simulink model "Induction_Motor_Simulation"  (R2021b)
settings: Solver=ode45  StartTime=0.0  StopTime=1  MinStep=1e-5  RelTol=1e-6
undefined symbols (not defined in the file): B, f_supply, J, L_ms, Lr_diag, Lr_non_diag, Ls_diag, Ls_non_diag, P, r_r, r_s, T_L, V_as, V_bs, V_cs
settings Model: Creator=pghat  LastModifiedBy=pghat
settings DebuggingCC: AlgebraicLoopMsg=none

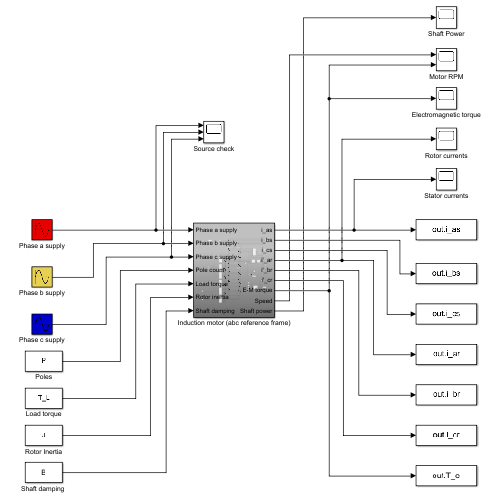
[thumbnail: Simulink's stored preview of the top-level diagram]
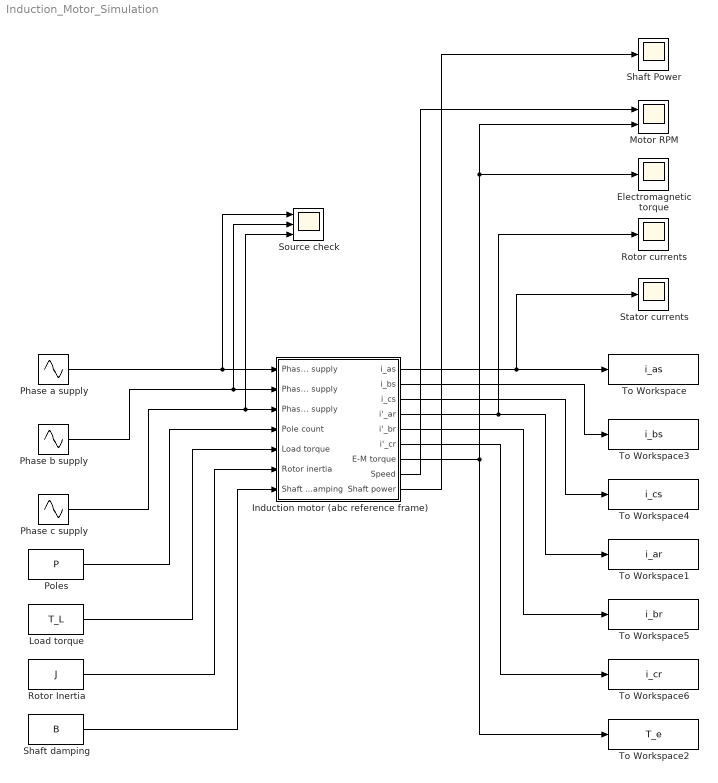
== system Induction_Motor_Simulation ==
  Electromagnetic torque : Scope
  Induction motor (abc reference frame) : Subsystem
  Load torque : Constant  Value=T_L
  Motor RPM : Scope  NumInputPorts=2
  Phase a supply : Sin  Amplitude=V_as  Frequency=f_supply  Phase=pi/2  SampleTime=0
  Phase b supply : Sin  Amplitude=V_bs  Frequency=f_supply  Phase=((2*pi)/3)+(pi/2)  SampleTime=0
  Phase c supply : Sin  Amplitude=V_cs  Frequency=f_supply  Phase=(-(2*pi)/3)+(pi/2)  SampleTime=0
  Poles : Constant  Value=P
  Rotor Inertia : Constant  Value=J
  Rotor currents : Scope
  Shaft Power : Scope
  "Shaft damping " : Constant  Value=B
  Source check : Scope  NumInputPorts=3
  Stator currents : Scope
  To Workspace : ToWorkspace  VariableName=i_as  SampleTime=-1
  To Workspace1 : ToWorkspace  VariableName=i_ar  SampleTime=-1
  To Workspace2 : ToWorkspace  VariableName=T_e  SampleTime=-1
  To Workspace3 : ToWorkspace  VariableName=i_bs  SampleTime=-1
  To Workspace4 : ToWorkspace  VariableName=i_cs  SampleTime=-1
  To Workspace5 : ToWorkspace  VariableName=i_br  SampleTime=-1
  To Workspace6 : ToWorkspace  VariableName=i_cr  SampleTime=-1
  wires:
  Poles/1 -> Induction motor (abc reference frame)/4(Pole count)
  Induction motor (abc reference frame)/4(i'_ar) -> To Workspace1/1, Rotor currents/1
  Induction motor (abc reference frame)/1(i_as) -> To Workspace/1, Stator currents/1
  Induction motor (abc reference frame)/7(E-M torque) -> To Workspace2/1, Motor RPM/2, Electromagnetic torque/1
  Phase a supply/1 -> Source check/1, Induction motor (abc reference frame)/1(Phase a supply)
  Phase b supply/1 -> Source check/2, Induction motor (abc reference frame)/2(Phase b supply)
  Phase c supply/1 -> Source check/3, Induction motor (abc reference frame)/3(Phase c supply)
  Rotor Inertia/1 -> Induction motor (abc reference frame)/6(Rotor inertia)
  Induction motor (abc reference frame)/8(Speed) -> Motor RPM/1
  Load torque/1 -> Induction motor (abc reference frame)/5(Load torque)
  "Shaft damping "/1 -> Induction motor (abc reference frame)/7(Shaft damping)
  Induction motor (abc reference frame)/2(i_bs) -> To Workspace3/1
  Induction motor (abc reference frame)/3(i_cs) -> To Workspace4/1
  Induction motor (abc reference frame)/5(i'_br) -> To Workspace5/1
  Induction motor (abc reference frame)/6(i'_cr) -> To Workspace6/1
  Induction motor (abc reference frame)/9(Shaft power) -> Shaft Power/1

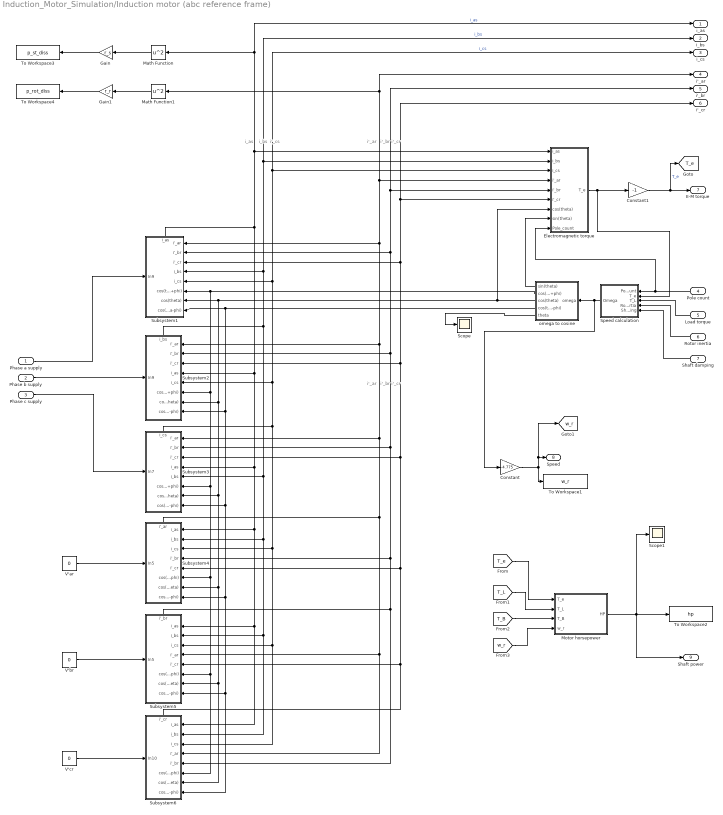
== system Induction_Motor_Simulation/Induction motor (abc reference frame) ==
  note: i'_ar
  note: i'_br
  note: i'_cr
  note: i_as
  note: i_bs
  note: i'_cs
  note: i'_br
  note: i'_ar
  note: i'_cr
  Phase a supply : Inport
  Phase b supply : Inport  Port=2
  Phase c supply : Inport  Port=3
  Pole count : Inport  Port=4
  Load torque : Inport  Port=5
  Rotor inertia : Inport  Port=6
  Shaft damping : Inport  Port=7
  Constant : Gain  Gain=-4.775
  Constant1 : Gain  Gain=-1
  Electromagnetic torque : Subsystem
  Gain : Gain  Gain=r_s
  Gain1 : Gain  Gain=r_r
  Math Function : Math  Operator=square  SaturateOnIntegerOverflow=on
  Math Function1 : Math  Operator=square  SaturateOnIntegerOverflow=on
  Motor horsepower : Subsystem
  Scope : Scope
  Scope1 : Scope
  Speed calculation : Subsystem
  Subsystem1 : Subsystem
      settings: PortSchema="{\"entries\":[{\"content\":{\"sides\":[{\"content\":{\"connectorIds\":[\"In1\",\"In2\",\"In3\",\"In4\",\"In5\",\"In6\",\"In7\",\"In8\"]},\"type\":\"ConnectorPlacement.EquallySpacedRectSide\",\"uuid\":\"ef07c968-7ee2-485d-9f10-a51b04dcb3ba\"},{\"content\":{\"connectorIds\":[\"In9\"],\"side\":\"RIGHT\"},\"type\":\"ConnectorPlacement.EquallySpacedRectSide\",\"uuid\":\"1cfd75a1-6326-417f-a91d-cffa3dd273c8\"},{\"content\":{\"connectorIds\":[\"Out1\"],\"side\":\"TOP\"},\"type\":\"ConnectorPlacement.EquallySpacedRectSide\",\"uuid\":\"a404849e-3712-479f-a728-f0b6851758dc\"}]},\"type\":\"ConnectorPlacement.EquallySpacedConnector\",\"uuid\":\"81e44c3d-c841-4212-bb95-4a45c20bd008\"}],\"packageUris\":[\"http://schema.mathworks.com/mf0/Connector/R2020b\"],\"version\":\"1.0\"}"
  Subsystem2 : Subsystem
      settings: PortSchema="{\"entries\":[{\"content\":{\"sides\":[{\"content\":{\"connectorIds\":[\"In1\",\"In2\",\"In3\",\"In4\",\"In5\",\"In6\",\"In7\",\"In8\"]},\"type\":\"ConnectorPlacement.EquallySpacedRectSide\",\"uuid\":\"ef07c968-7ee2-485d-9f10-a51b04dcb3ba\"},{\"content\":{\"connectorIds\":[\"In9\"],\"side\":\"RIGHT\"},\"type\":\"ConnectorPlacement.EquallySpacedRectSide\",\"uuid\":\"1cfd75a1-6326-417f-a91d-cffa3dd273c8\"},{\"content\":{\"connectorIds\":[\"Out1\"],\"side\":\"TOP\"},\"type\":\"ConnectorPlacement.EquallySpacedRectSide\",\"uuid\":\"a404849e-3712-479f-a728-f0b6851758dc\"}]},\"type\":\"ConnectorPlacement.EquallySpacedConnector\",\"uuid\":\"81e44c3d-c841-4212-bb95-4a45c20bd008\"}],\"packageUris\":[\"http://schema.mathworks.com/mf0/Connector/R2020b\"],\"version\":\"1.0\"}"
  Subsystem3 : Subsystem
      settings: PortSchema="{\"entries\":[{\"content\":{\"sides\":[{\"content\":{\"connectorIds\":[\"In1\",\"In2\",\"In3\",\"In4\",\"In5\",\"In6\",\"In7\",\"In8\"]},\"type\":\"ConnectorPlacement.EquallySpacedRectSide\",\"uuid\":\"ef07c968-7ee2-485d-9f10-a51b04dcb3ba\"},{\"content\":{\"connectorIds\":[\"In9\"],\"side\":\"RIGHT\"},\"type\":\"ConnectorPlacement.EquallySpacedRectSide\",\"uuid\":\"1cfd75a1-6326-417f-a91d-cffa3dd273c8\"},{\"content\":{\"connectorIds\":[\"Out1\"],\"side\":\"TOP\"},\"type\":\"ConnectorPlacement.EquallySpacedRectSide\",\"uuid\":\"a404849e-3712-479f-a728-f0b6851758dc\"}]},\"type\":\"ConnectorPlacement.EquallySpacedConnector\",\"uuid\":\"81e44c3d-c841-4212-bb95-4a45c20bd008\"}],\"packageUris\":[\"http://schema.mathworks.com/mf0/Connector/R2020b\"],\"version\":\"1.0\"}"
  Subsystem4 : Subsystem
      settings: PortSchema="{\"entries\":[{\"content\":{\"sides\":[{\"content\":{\"connectorIds\":[\"In1\",\"In2\",\"In3\",\"In4\",\"In5\",\"In6\",\"In7\",\"In8\"]},\"type\":\"ConnectorPlacement.EquallySpacedRectSide\",\"uuid\":\"ef07c968-7ee2-485d-9f10-a51b04dcb3ba\"},{\"content\":{\"connectorIds\":[\"In9\"],\"side\":\"RIGHT\"},\"type\":\"ConnectorPlacement.EquallySpacedRectSide\",\"uuid\":\"1cfd75a1-6326-417f-a91d-cffa3dd273c8\"},{\"content\":{\"connectorIds\":[\"Out1\"],\"side\":\"TOP\"},\"type\":\"ConnectorPlacement.EquallySpacedRectSide\",\"uuid\":\"a404849e-3712-479f-a728-f0b6851758dc\"}]},\"type\":\"ConnectorPlacement.EquallySpacedConnector\",\"uuid\":\"81e44c3d-c841-4212-bb95-4a45c20bd008\"}],\"packageUris\":[\"http://schema.mathworks.com/mf0/Connector/R2020b\"],\"version\":\"1.0\"}"
  Subsystem5 : Subsystem
      settings: PortSchema="{\"entries\":[{\"content\":{\"sides\":[{\"content\":{\"connectorIds\":[\"In1\",\"In2\",\"In3\",\"In4\",\"In5\",\"In6\",\"In7\",\"In8\"]},\"type\":\"ConnectorPlacement.EquallySpacedRectSide\",\"uuid\":\"0210d93f-9c3f-4c48-b905-c827d03e93dd\"},{\"content\":{\"connectorIds\":[\"In9\"],\"side\":\"RIGHT\"},\"type\":\"ConnectorPlacement.EquallySpacedRectSide\",\"uuid\":\"c736d190-453a-4343-8a19-c27848e7902e\"},{\"content\":{\"connectorIds\":[\"Out1\"],\"side\":\"TOP\"},\"type\":\"ConnectorPlacement.EquallySpacedRectSide\",\"uuid\":\"5fb2e819-973b-468f-b715-ca8a0cef9cb3\"},{\"content\":{\"connectorIds\":[],\"side\":\"BOTTOM\"},\"type\":\"ConnectorPlacement.EquallySpacedRectSide\",\"uuid\":\"5f03be8f-1406-459f-bd04-ec8e4d38f84a\"}]},\"type\":\"ConnectorPlacement.EquallySpacedConnector\",\"uuid\":\"f8abb9ea-f237-42db-8404-f45f7fcbb037\"}],\"packageUris\":[\"http://schema.mathworks.com/mf0/Connector/R2020b\"],\"version\":\"1.0\"}"
  Subsystem6 : Subsystem
      settings: PortSchema="{\"entries\":[{\"content\":{\"sides\":[{\"content\":{\"connectorIds\":[\"In1\",\"In2\",\"In3\",\"In4\",\"In5\",\"In6\",\"In7\",\"In8\"]},\"type\":\"ConnectorPlacement.EquallySpacedRectSide\",\"uuid\":\"0210d93f-9c3f-4c48-b905-c827d03e93dd\"},{\"content\":{\"connectorIds\":[\"In9\"],\"side\":\"RIGHT\"},\"type\":\"ConnectorPlacement.EquallySpacedRectSide\",\"uuid\":\"c736d190-453a-4343-8a19-c27848e7902e\"},{\"content\":{\"connectorIds\":[\"Out1\"],\"side\":\"TOP\"},\"type\":\"ConnectorPlacement.EquallySpacedRectSide\",\"uuid\":\"5fb2e819-973b-468f-b715-ca8a0cef9cb3\"}]},\"type\":\"ConnectorPlacement.EquallySpacedConnector\",\"uuid\":\"f8abb9ea-f237-42db-8404-f45f7fcbb037\"}],\"packageUris\":[\"http://schema.mathworks.com/mf0/Connector/R2020b\"],\"version\":\"1.0\"}"
  To Workspace1 : ToWorkspace  VariableName=w_r  SampleTime=-1
  To Workspace2 : ToWorkspace  VariableName=hp  SampleTime=-1
  To Workspace3 : ToWorkspace  VariableName=p_st_diss  SampleTime=-1
  To Workspace4 : ToWorkspace  VariableName=p_rot_diss  SampleTime=-1
  V'ar : Constant  Value=0
  V'br : Constant  Value=0
  V'cr : Constant  Value=0
  omega to cosine : Subsystem
  i_as : Outport
  i_bs : Outport  Port=2
  i_cs : Outport  Port=3
  i'_ar : Outport  Port=4
  i'_br : Outport  Port=5
  i'_cr : Outport  Port=6
  E-M torque : Outport  Port=7
  Speed : Outport  Port=8
  Shaft power : Outport  Port=9
  tag scope: T_e=global, w_r=global
  wires:
  omega to cosine/1(sin(theta)) -> Electromagnetic torque/8(sin(theta))
  Pole count/1 -> Electromagnetic torque/9(Pole_count), Speed calculation/1(Pole count)
  Electromagnetic torque/1(T_e) -> Speed calculation/2(T_e), Constant1/1
  Constant1/1 -> [T_e], E-M torque/1  "T_e"
  Speed calculation/1(Omega) -> Constant/1, omega to cosine/1(omega)
  Constant/1 -> Speed/1, [w_r], To Workspace1/1
  Rotor inertia/1 -> Speed calculation/4(Rotor Inertia)
  Phase a supply/1 -> Subsystem1/9(In9)
  Phase b supply/1 -> Subsystem2/9(In9)
  Phase c supply/1 -> Subsystem3/9(In7)
  V'ar/1 -> Subsystem4/9(In5)
  V'br/1 -> Subsystem5/9(In5)
  V'cr/1 -> Subsystem6/9(In10)
  Subsystem1/1(i_as) -> Math Function/1, i_as/1, Electromagnetic torque/1(i_as), Subsystem6/1(i_as), Subsystem5/1(i_as), Subsystem4/1(i_as), Subsystem3/4(i_as), Subsystem2/4(i_as)  "i_as"
  Subsystem2/1(i_bs) -> i_bs/1, Electromagnetic torque/2(i_bs), Subsystem1/4(i_bs), Subsystem6/2(i_bs), Subsystem5/2(i_bs), Subsystem4/2(i_bs), Subsystem3/5(i_bs)  "i_bs"
  Subsystem3/1(i_cs) -> Subsystem6/3(i_cs), Subsystem5/3(i_cs), Subsystem4/3(i_cs), i_cs/1, Electromagnetic torque/3(i_cs), Subsystem1/5(i_cs), Subsystem2/5(i_cs)  "i_cs"
  Subsystem5/1(i'_br) -> i'_br/1, Electromagnetic torque/5(i'_br), Subsystem1/2(i'_br), Subsystem2/2(i'_br), Subsystem3/2(i'_br), Subsystem4/4(i'_br), Subsystem6/5(i'_br)
  omega to cosine/2(cos(theta+phi)) -> Subsystem6/6(cos(theta+phi)), Subsystem5/6(cos(theta+phi)), Subsystem4/6(cos(theta+phi)), Subsystem3/6(cos(theta+phi)), Subsystem2/6(cos(theta+phi)), Subsystem1/6(cos(theta+phi))
  omega to cosine/3(cos(theta)) -> Electromagnetic torque/7(cos(theta)), Subsystem5/7(cos(theta)), Subsystem6/7(cos(theta)), Subsystem4/7(cos(theta)), Subsystem3/7(cos(theta)), Subsystem2/7(cos(theta)), Subsystem1/7(cos(theta))
  omega to cosine/4(cos(theta-phi)) -> Subsystem6/8(cos(theta-phi)), Subsystem5/8(cos(theta-phi)), Subsystem4/8(cos(theta-phi)), Subsystem3/8(cos(theta-phi)), Subsystem2/8(cos(theta-phi)), Subsystem1/8(cos(theta-phi))
  Subsystem4/1(i'_ar) -> Math Function1/1, i'_ar/1, Electromagnetic torque/4(i'_ar), Subsystem1/1(i'_ar), Subsystem2/1(i'_ar), Subsystem3/1(i'_ar), Subsystem6/4(i'_ar), Subsystem5/4(i'_ar)
  Subsystem6/1(i'_cr) -> Subsystem5/5(i'_cr), i'_cr/1, Electromagnetic torque/6(i'_cr), Subsystem1/3(i'_cr), Subsystem2/3(i'_cr), Subsystem3/3(i'_cr), Subsystem4/5(i'_cr)
  omega to cosine/5(theta) -> Scope/1
  Shaft damping/1 -> Speed calculation/5(Shaft damping)
  Load torque/1 -> Speed calculation/3(T_L)
  [T_e] -> Motor horsepower/1(T_e)
  [T_L] -> Motor horsepower/2(T_L)
  [T_B] -> Motor horsepower/3(T_B)
  [w_r] -> Motor horsepower/4(w_r)
  Motor horsepower/1(HP) -> Shaft power/1, To Workspace2/1, Scope1/1
  Math Function/1 -> Gain/1
  Math Function1/1 -> Gain1/1
  Gain/1 -> To Workspace3/1
  Gain1/1 -> To Workspace4/1

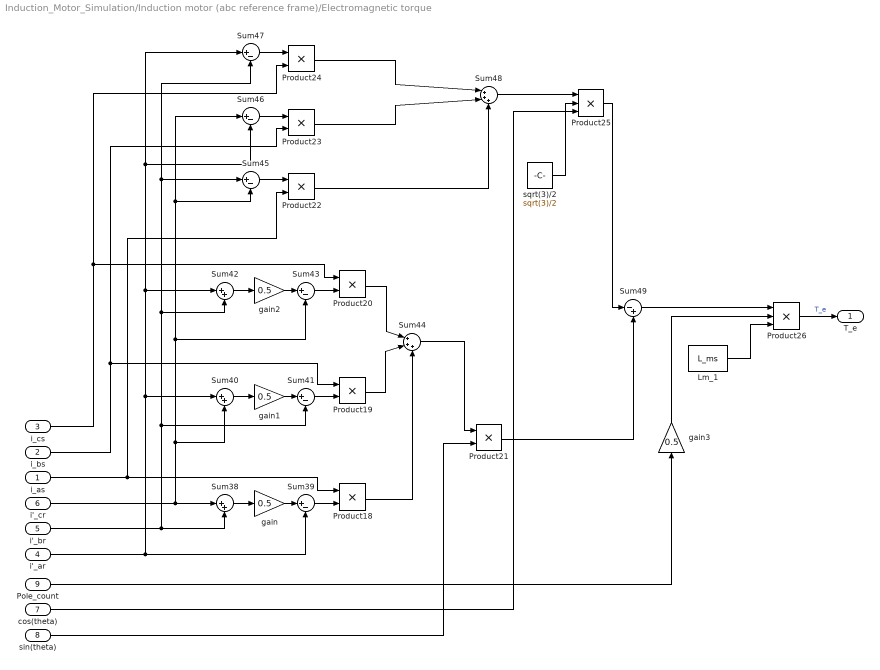
== system Induction_Motor_Simulation/Induction motor (abc reference frame)/Electromagnetic torque ==
  i_as : Inport
  i_bs : Inport  Port=2
  i_cs : Inport  Port=3
  i'_ar : Inport  Port=4
  i'_br : Inport  Port=5
  i'_cr : Inport  Port=6
  cos(theta) : Inport  Port=7
  sin(theta) : Inport  Port=8
  Pole_count : Inport  Port=9
  Lm_1 : Constant  Value=L_ms
  Product{18..24} (7 alike) : Product
  Product25 : Product  Inputs=3
  Product26 : Product  Inputs=3
  Sum38 : Sum  Inputs=|++
  Sum{39,41,43,45..47} (6 alike) : Sum  Inputs=|+-
  Sum40 : Sum  Inputs=|++
  Sum42 : Sum  Inputs=|++
  Sum44 : Sum  Inputs=|+++
  Sum48 : Sum  Inputs=|+++
  Sum49 : Sum  Inputs=|-+
  gain{,1..3} (4 alike) : Gain  Gain=0.5
  sqrt(3)/2 : Constant  Value=sqrt(3)/2
  T_e : Outport
  wires:
  gain/1 -> Sum39/1
  Sum40/1 -> gain1/1
  i_bs/1 -> Product23/2, Product19/1
  Product25/1 -> Sum49/1
  Product24/1 -> Sum48/1
  gain1/1 -> Sum41/1
  Sum46/1 -> Product23/1
  cos(theta)/1 -> Product25/3
  Sum44/1 -> Product21/1
  Sum43/1 -> Product20/2
  Sum38/1 -> gain/1
  Product23/1 -> Sum48/2
  i'_br/1 -> Sum41/2, Sum47/2, Sum45/1, Sum42/2, Sum38/2
  Sum47/1 -> Product24/1
  sin(theta)/1 -> Product21/2
  i'_ar/1 -> Sum40/1, Sum42/1, Sum47/1, Sum46/2, Sum39/2
  i'_cr/1 -> Sum38/1, Sum40/2, Sum46/1, Sum45/2, Sum43/2
  Sum49/1 -> Product26/1
  Product18/1 -> Sum44/3
  i_as/1 -> Product22/2, Product18/1
  Lm_1/1 -> Product26/3
  Sum45/1 -> Product22/1
  Product26/1 -> T_e/1  "T_e"
  Product19/1 -> Sum44/2
  Product20/1 -> Sum44/1
  Sum42/1 -> gain2/1
  sqrt(3)/2/1 -> Product25/2
  Sum41/1 -> Product19/2
  Product22/1 -> Sum48/3
  Product21/1 -> Sum49/2
  i_cs/1 -> Product20/1, Product24/2
  Sum48/1 -> Product25/1
  Sum39/1 -> Product18/2
  gain2/1 -> Sum43/1
  gain3/1 -> Product26/2
  Pole_count/1 -> gain3/1

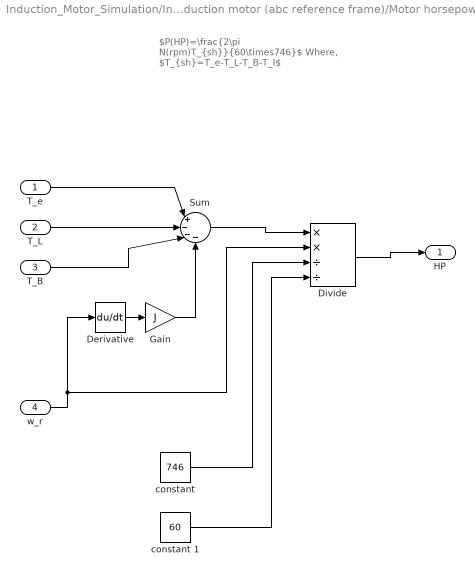
== system Induction_Motor_Simulation/Induction motor (abc reference frame)/Motor horsepower ==
  note: $P(HP)=\frac{2\pi N(rpm)T_{sh}}{60\times746}$
      | Where,
      |
      | $T_{sh}=T_e-T_L-T_B-T_I$
  T_e : Inport
  T_L : Inport  Port=2
  T_B : Inport  Port=3
  w_r : Inport  Port=4
  Derivative : Derivative
  Divide : Product  Inputs=**//
  Gain : Gain  Gain=J
  Sum : Sum  Inputs=|+---
  "constant " : Constant  Value=746
  constant 1 : Constant  Value=60
  HP : Outport
  wires:
  T_B/1 -> Sum/3
  Sum/1 -> Divide/1
  T_L/1 -> Sum/2
  T_e/1 -> Sum/1
  Divide/1 -> HP/1
  w_r/1 -> Derivative/1, Divide/2
  "constant "/1 -> Divide/3
  Derivative/1 -> Gain/1
  Gain/1 -> Sum/4
  constant 1/1 -> Divide/4

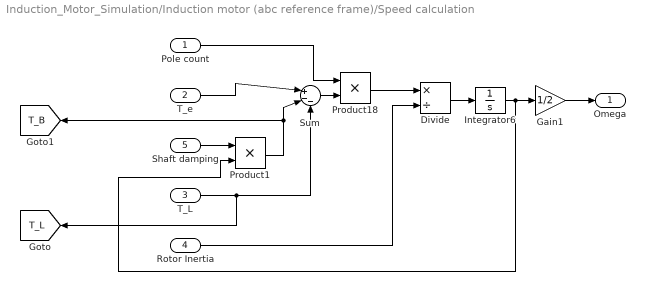
== system Induction_Motor_Simulation/Induction motor (abc reference frame)/Speed calculation ==
  Pole count : Inport
  T_e : Inport  Port=2
  T_L : Inport  Port=3
  Rotor Inertia : Inport  Port=4
  Shaft damping : Inport  Port=5
  Divide : Product  Inputs=*/
  Gain1 : Gain  Gain=1/2
  Integrator6 : Integrator  UpperSaturationLimit=-inf
  Product1 : Product
  Product18 : Product
  Sum : Sum  Inputs=|+--
  Omega : Outport
  tag scope: T_B=global, T_L=global
  wires:
  Rotor Inertia/1 -> Divide/2
  Product18/1 -> Divide/1
  Divide/1 -> Integrator6/1
  Integrator6/1 -> Gain1/1, Product1/2
  T_e/1 -> Sum/1
  Sum/1 -> Product18/2
  T_L/1 -> [T_L], Sum/3
  Shaft damping/1 -> Product1/1
  Product1/1 -> [T_B], Sum/2
  Gain1/1 -> Omega/1
  Pole count/1 -> Product18/1

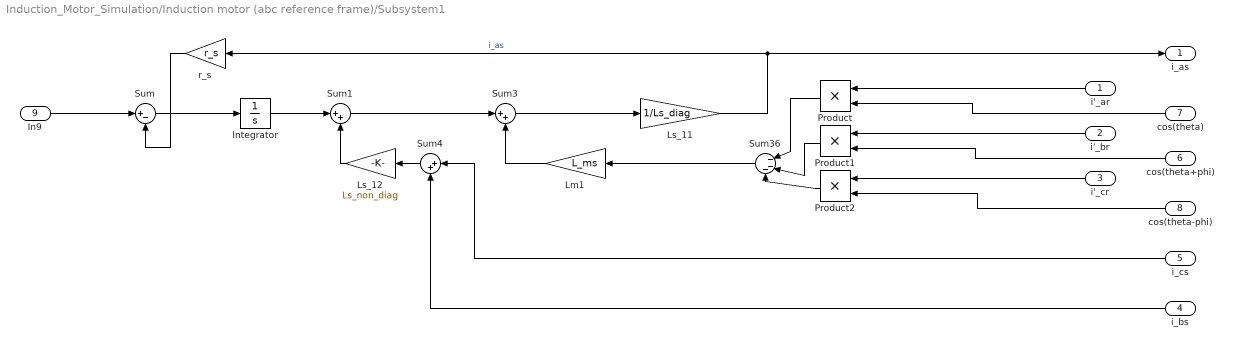
== system Induction_Motor_Simulation/Induction motor (abc reference frame)/Subsystem1 ==
  i'_ar : Inport
  i'_br : Inport  Port=2
  i'_cr : Inport  Port=3
  i_bs : Inport  Port=4
  i_cs : Inport  Port=5
  cos(theta+phi) : Inport  Port=6
  cos(theta) : Inport  Port=7
  cos(theta-phi) : Inport  Port=8
  In9 : Inport  Port=9
  Integrator : Integrator
  Lm1 : Gain  Gain=L_ms
  Ls_11 : Gain  Gain=1/Ls_diag
  Ls_12 : Gain  Gain=Ls_non_diag
  Product : Product
  Product1 : Product
  Product2 : Product
  Sum : Sum  Inputs=|+-
  Sum1 : Sum  Inputs=|++
  Sum3 : Sum  Inputs=|++
  Sum36 : Sum  Inputs=|---
  Sum4 : Sum  Inputs=|++
  r_s : Gain  Gain=r_s
  i_as : Outport
  wires:
  Product/1 -> Sum36/1
  cos(theta+phi)/1 -> Product1/2
  Sum4/1 -> Ls_12/1
  i'_ar/1 -> Product/1
  Sum1/1 -> Sum3/1
  Sum/1 -> Integrator/1
  Ls_11/1 -> i_as/1, r_s/1  "i_as"
  Ls_12/1 -> Sum1/2
  cos(theta-phi)/1 -> Product2/2
  Product1/1 -> Sum36/2
  r_s/1 -> Sum/2
  Sum36/1 -> Lm1/1
  Product2/1 -> Sum36/3
  Sum3/1 -> Ls_11/1
  Lm1/1 -> Sum3/2
  Integrator/1 -> Sum1/1
  cos(theta)/1 -> Product/2
  i'_br/1 -> Product1/1
  i_bs/1 -> Sum4/2
  In9/1 -> Sum/1
  i'_cr/1 -> Product2/1
  i_cs/1 -> Sum4/1

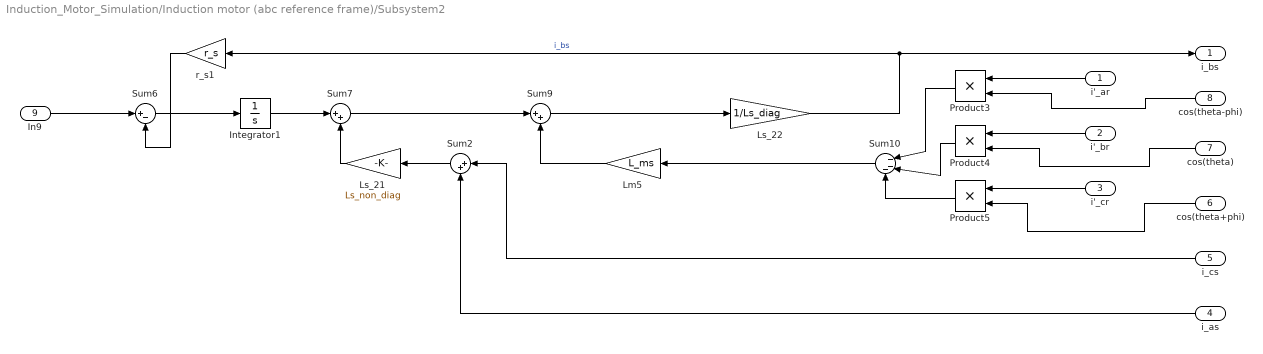
== system Induction_Motor_Simulation/Induction motor (abc reference frame)/Subsystem2 ==
  i'_ar : Inport
  i'_br : Inport  Port=2
  i'_cr : Inport  Port=3
  i_as : Inport  Port=4
  i_cs : Inport  Port=5
  cos(theta+phi) : Inport  Port=6
  cos(theta) : Inport  Port=7
  cos(theta-phi) : Inport  Port=8
  In9 : Inport  Port=9
  Integrator1 : Integrator
  Lm5 : Gain  Gain=L_ms
  Ls_21 : Gain  Gain=Ls_non_diag
  Ls_22 : Gain  Gain=1/Ls_diag
  Product3 : Product
  Product4 : Product
  Product5 : Product
  Sum10 : Sum  Inputs=|---
  Sum2 : Sum  Inputs=|++
  Sum6 : Sum  Inputs=|+-
  Sum7 : Sum  Inputs=|++
  Sum9 : Sum  Inputs=|++
  r_s1 : Gain  Gain=r_s
  i_bs : Outport
  wires:
  i_cs/1 -> Sum2/1
  Lm5/1 -> Sum9/2
  Ls_22/1 -> i_bs/1, r_s1/1  "i_bs"
  Sum6/1 -> Integrator1/1
  Sum7/1 -> Sum9/1
  Sum9/1 -> Ls_22/1
  r_s1/1 -> Sum6/2
  Ls_21/1 -> Sum7/2
  Product4/1 -> Sum10/2
  Sum2/1 -> Ls_21/1
  Product3/1 -> Sum10/1
  i'_ar/1 -> Product3/1
  Sum10/1 -> Lm5/1
  Product5/1 -> Sum10/3
  Integrator1/1 -> Sum7/1
  i'_br/1 -> Product4/1
  i'_cr/1 -> Product5/1
  i_as/1 -> Sum2/2
  In9/1 -> Sum6/1
  cos(theta+phi)/1 -> Product5/2
  cos(theta-phi)/1 -> Product3/2
  cos(theta)/1 -> Product4/2

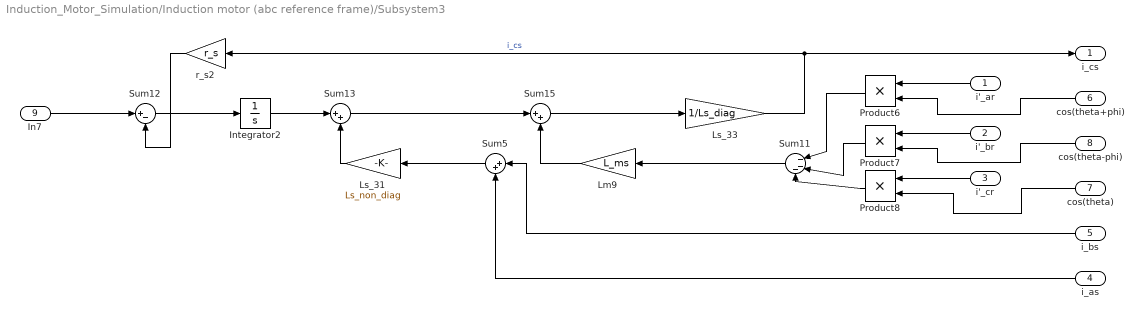
== system Induction_Motor_Simulation/Induction motor (abc reference frame)/Subsystem3 ==
  i'_ar : Inport
  i'_br : Inport  Port=2
  i'_cr : Inport  Port=3
  i_as : Inport  Port=4
  i_bs : Inport  Port=5
  cos(theta+phi) : Inport  Port=6
  cos(theta) : Inport  Port=7
  cos(theta-phi) : Inport  Port=8
  In7 : Inport  Port=9
  Integrator2 : Integrator
  Lm9 : Gain  Gain=L_ms
  Ls_31 : Gain  Gain=Ls_non_diag
  Ls_33 : Gain  Gain=1/Ls_diag
  Product6 : Product
  Product7 : Product
  Product8 : Product
  Sum11 : Sum  Inputs=|---
  Sum12 : Sum  Inputs=|+-
  Sum13 : Sum  Inputs=|++
  Sum15 : Sum  Inputs=|++
  Sum5 : Sum  Inputs=|++
  r_s2 : Gain  Gain=r_s
  i_cs : Outport
  wires:
  Product8/1 -> Sum11/3
  Sum12/1 -> Integrator2/1
  cos(theta)/1 -> Product8/2
  Product7/1 -> Sum11/2
  Ls_31/1 -> Sum13/2
  r_s2/1 -> Sum12/2
  Sum15/1 -> Ls_33/1
  Product6/1 -> Sum11/1
  Lm9/1 -> Sum15/2
  Sum11/1 -> Lm9/1
  Ls_33/1 -> r_s2/1, i_cs/1  "i_cs"
  Integrator2/1 -> Sum13/1
  Sum13/1 -> Sum15/1
  Sum5/1 -> Ls_31/1
  i'_br/1 -> Product7/1
  i'_ar/1 -> Product6/1
  i_bs/1 -> Sum5/1
  In7/1 -> Sum12/1
  i'_cr/1 -> Product8/1
  i_as/1 -> Sum5/2
  cos(theta+phi)/1 -> Product6/2
  cos(theta-phi)/1 -> Product7/2

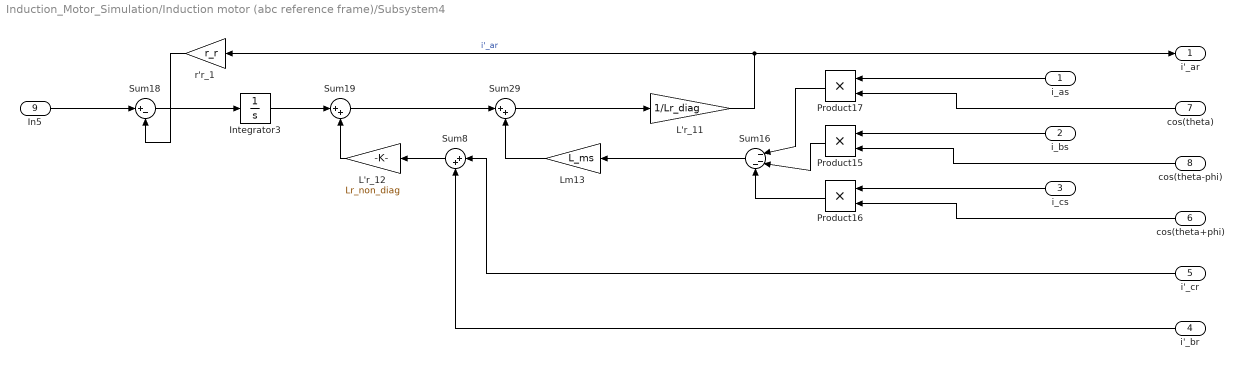
== system Induction_Motor_Simulation/Induction motor (abc reference frame)/Subsystem4 ==
  i_as : Inport
  i_bs : Inport  Port=2
  i_cs : Inport  Port=3
  i'_br : Inport  Port=4
  i'_cr : Inport  Port=5
  cos(theta+phi) : Inport  Port=6
  cos(theta) : Inport  Port=7
  cos(theta-phi) : Inport  Port=8
  In5 : Inport  Port=9
  Integrator3 : Integrator
  L'r_11 : Gain  Gain=1/Lr_diag
  L'r_12 : Gain  Gain=Lr_non_diag
  Lm13 : Gain  Gain=L_ms
  Product15 : Product
  Product16 : Product
  Product17 : Product
  Sum16 : Sum  Inputs=|---
  Sum18 : Sum  Inputs=|+-
  Sum19 : Sum  Inputs=|++
  Sum29 : Sum  Inputs=|++
  Sum8 : Sum  Inputs=|++
  r'r_1 : Gain  Gain=r_r
  i'_ar : Outport
  wires:
  Product17/1 -> Sum16/1
  Integrator3/1 -> Sum19/1
  L'r_11/1 -> r'r_1/1, i'_ar/1  "i'_ar"
  r'r_1/1 -> Sum18/2
  Sum18/1 -> Integrator3/1
  i_cs/1 -> Product16/1
  Product16/1 -> Sum16/3
  Lm13/1 -> Sum29/2
  Sum16/1 -> Lm13/1
  cos(theta+phi)/1 -> Product16/2
  i'_cr/1 -> Sum8/1
  Sum29/1 -> L'r_11/1
  Sum8/1 -> L'r_12/1
  Product15/1 -> Sum16/2
  Sum19/1 -> Sum29/1
  i_as/1 -> Product17/1
  In5/1 -> Sum18/1
  L'r_12/1 -> Sum19/2
  i'_br/1 -> Sum8/2
  i_bs/1 -> Product15/1
  cos(theta)/1 -> Product17/2
  cos(theta-phi)/1 -> Product15/2

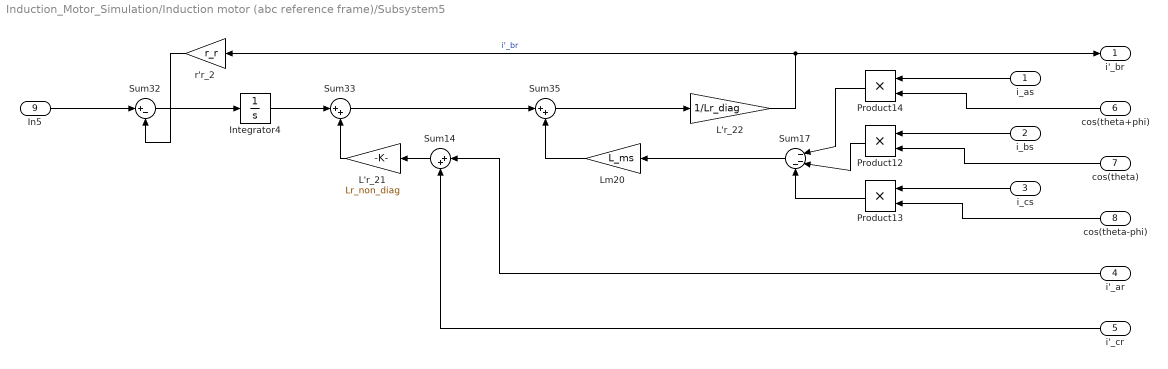
== system Induction_Motor_Simulation/Induction motor (abc reference frame)/Subsystem5 ==
  i_as : Inport
  i_bs : Inport  Port=2
  i_cs : Inport  Port=3
  i'_ar : Inport  Port=4
  i'_cr : Inport  Port=5
  cos(theta+phi) : Inport  Port=6
  cos(theta) : Inport  Port=7
  cos(theta-phi) : Inport  Port=8
  In5 : Inport  Port=9
  Integrator4 : Integrator
  L'r_21 : Gain  Gain=Lr_non_diag
  L'r_22 : Gain  Gain=1/Lr_diag
  Lm20 : Gain  Gain=L_ms
  Product12 : Product
  Product13 : Product
  Product14 : Product
  Sum14 : Sum  Inputs=|++
  Sum17 : Sum  Inputs=|---
  Sum32 : Sum  Inputs=|+-
  Sum33 : Sum  Inputs=|++
  Sum35 : Sum  Inputs=|++
  r'r_2 : Gain  Gain=r_r
  i'_br : Outport
  wires:
  L'r_21/1 -> Sum33/2
  Sum35/1 -> L'r_22/1
  Product13/1 -> Sum17/3
  Lm20/1 -> Sum35/2
  In5/1 -> Sum32/1
  Integrator4/1 -> Sum33/1
  Sum32/1 -> Integrator4/1
  r'r_2/1 -> Sum32/2
  Product12/1 -> Sum17/2
  Sum17/1 -> Lm20/1
  Sum14/1 -> L'r_21/1
  Product14/1 -> Sum17/1
  Sum33/1 -> Sum35/1
  i_cs/1 -> Product13/1
  cos(theta-phi)/1 -> Product13/2
  i'_ar/1 -> Sum14/1
  L'r_22/1 -> r'r_2/1, i'_br/1  "i'_br"
  i_bs/1 -> Product12/1
  i'_cr/1 -> Sum14/2
  i_as/1 -> Product14/1
  cos(theta)/1 -> Product12/2
  cos(theta+phi)/1 -> Product14/2

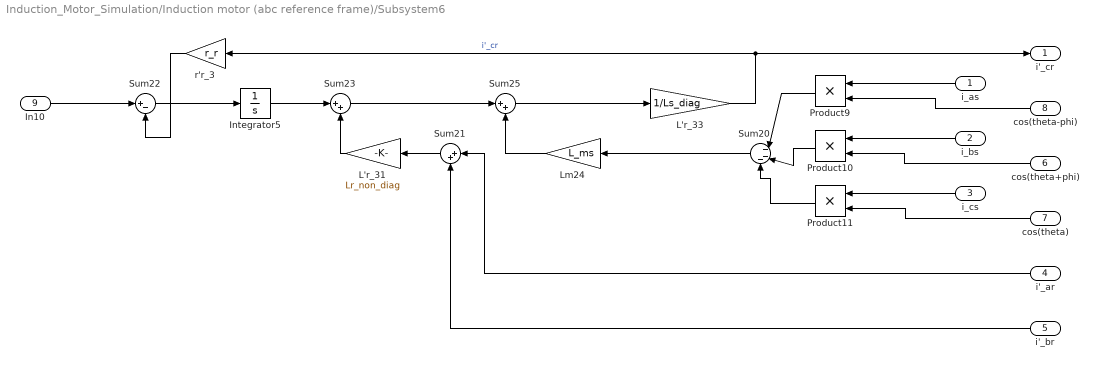
== system Induction_Motor_Simulation/Induction motor (abc reference frame)/Subsystem6 ==
  i_as : Inport
  i_bs : Inport  Port=2
  i_cs : Inport  Port=3
  i'_ar : Inport  Port=4
  i'_br : Inport  Port=5
  cos(theta+phi) : Inport  Port=6
  cos(theta) : Inport  Port=7
  cos(theta-phi) : Inport  Port=8
  In10 : Inport  Port=9
  Integrator5 : Integrator
  L'r_31 : Gain  Gain=Lr_non_diag
  L'r_33 : Gain  Gain=1/Ls_diag
  Lm24 : Gain  Gain=L_ms
  Product10 : Product
  Product11 : Product
  Product9 : Product
  Sum20 : Sum  Inputs=|---
  Sum21 : Sum  Inputs=|++
  Sum22 : Sum  Inputs=|+-
  Sum23 : Sum  Inputs=|++
  Sum25 : Sum  Inputs=|++
  r'r_3 : Gain  Gain=r_r
  i'_cr : Outport
  wires:
  L'r_33/1 -> r'r_3/1, i'_cr/1  "i'_cr"
  i'_ar/1 -> Sum21/1
  Integrator5/1 -> Sum23/1
  Product10/1 -> Sum20/2
  Sum22/1 -> Integrator5/1
  L'r_31/1 -> Sum23/2
  i_as/1 -> Product9/1
  Sum20/1 -> Lm24/1
  cos(theta+phi)/1 -> Product10/2
  Lm24/1 -> Sum25/2
  In10/1 -> Sum22/1
  i_cs/1 -> Product11/1
  Sum21/1 -> L'r_31/1
  Sum23/1 -> Sum25/1
  r'r_3/1 -> Sum22/2
  cos(theta)/1 -> Product11/2
  Product9/1 -> Sum20/1
  Product11/1 -> Sum20/3
  Sum25/1 -> L'r_33/1
  cos(theta-phi)/1 -> Product9/2
  i_bs/1 -> Product10/1
  i'_br/1 -> Sum21/2

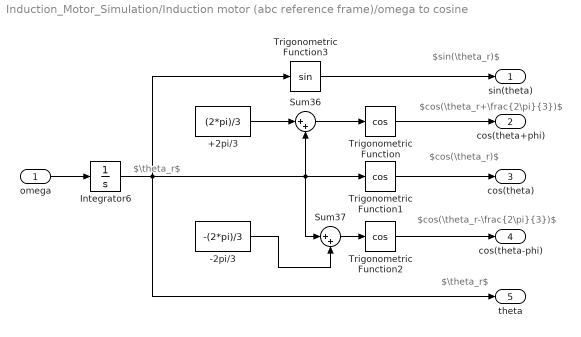
== system Induction_Motor_Simulation/Induction motor (abc reference frame)/omega to cosine ==
  note: $cos(\theta_r+\frac{2\pi}{3})$
  note: $cos(\theta_r-\frac{2\pi}{3})$
  note: $cos(\theta_r)$
  note: $sin(\theta_r)$
  note: $\theta_r$
  note: $\theta_r$
  omega : Inport
  +2pi/3 : Constant  Value=(2*pi)/3  VectorParams1D=off
  -2pi/3 : Constant  Value=-(2*pi)/3
  Integrator6 : Integrator
  Sum36 : Sum  Inputs=|++
  Sum37 : Sum  Inputs=|++
  Trigonometric Function : Trigonometry  Operator=cos
  Trigonometric Function1 : Trigonometry  Operator=cos
  Trigonometric Function2 : Trigonometry  Operator=cos
  Trigonometric Function3 : Trigonometry
  sin(theta) : Outport
  cos(theta+phi) : Outport  Port=2
  cos(theta) : Outport  Port=3
  cos(theta-phi) : Outport  Port=4
  theta : Outport  Port=5
  wires:
  Integrator6/1 -> Sum37/1, Trigonometric Function1/1, Sum36/2, theta/1, Trigonometric Function3/1
  Trigonometric Function3/1 -> sin(theta)/1
  -2pi/3/1 -> Sum37/2
  Trigonometric Function1/1 -> cos(theta)/1
  Sum36/1 -> Trigonometric Function/1
  Trigonometric Function/1 -> cos(theta+phi)/1
  +2pi/3/1 -> Sum36/1
  Sum37/1 -> Trigonometric Function2/1
  Trigonometric Function2/1 -> cos(theta-phi)/1
  omega/1 -> Integrator6/1
